simulink model "SITL"  (R2018a)
settings: Solver=VariableStepAuto  StartTime=0.0  StopTime=1000  RelTol=1e-3
settings Model: Creator=Usuario  LastModifiedBy=Usuario

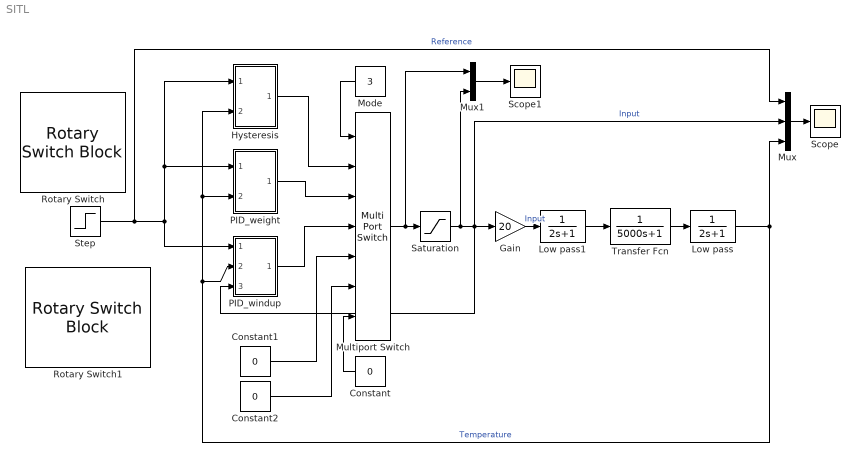
== system SITL ==
  Constant : Constant  Value=0
  Constant1 : Constant  Value=0
  Constant2 : Constant  Value=0
  Gain : Gain  Gain=20
  Hysteresis : Subsystem
  Low pass : TransferFcn  Denominator=[2 1]
  Low pass1 : TransferFcn  Denominator=[2 1]
  Mode : Constant  Value=3
  Multiport Switch : MultiPortSwitch  Inputs=5  DataPortForDefault=Additional data port
  Mux : Mux  Inputs=3
  Mux1 : Mux  Inputs=2
  PID_weight : Subsystem
  PID_windup : Subsystem
  Rotary Switch : RotarySwitchBlock  WebBlockId=48  LabelPosition=Bottom
      settings: Values={{'Off', 'Δ10', 'Δ30', 'Δ50'}, [0 10 30 50]}
  Rotary Switch1 : RotarySwitchBlock  WebBlockId=49  LabelPosition=Bottom
      settings: Values={{'Hyst', 'weight', 'windup', 'filter', 'Events'}, [1 2 3 4 5]}
  Saturation : Saturate  UpperLimit=100  LowerLimit=0
  Scope : Scope
  Scope1 : Scope
  Step : Step  Time=0  After=50  SampleTime=0
  Transfer Fcn : TransferFcn  Denominator=[5000 1]
  wires:
  Step/1 -> Mux/1, Hysteresis/1(Reference), PID_weight/1(Reference), PID_windup/1(Reference)  "Reference"
  Transfer Fcn/1 -> Low pass/1
  Mux/1 -> Scope/1
  Saturation/1 -> Mux1/2, PID_windup/3(Saturated), Mux/2, Gain/1  "Input"
  Multiport Switch/1 -> Mux1/1, Saturation/1
  Low pass/1 -> PID_windup/2(State), PID_weight/2(State), Hysteresis/2(State), Mux/3  "Temperature"
  Gain/1 -> Low pass1/1  "Input"
  Low pass1/1 -> Transfer Fcn/1
  Constant/1 -> Multiport Switch/7
  Hysteresis/1(Out) -> Multiport Switch/2
  PID_weight/1(Out) -> Multiport Switch/3
  Mode/1 -> Multiport Switch/1
  PID_windup/1(Out) -> Multiport Switch/4
  Mux1/1 -> Scope1/1
  Constant1/1 -> Multiport Switch/5
  Constant2/1 -> Multiport Switch/6

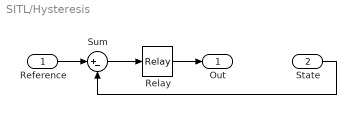
== system SITL/Hysteresis ==
  Reference : Inport
  State : Inport  Port=2
  Relay : Relay  OnSwitchValue=2  OffSwitchValue=0  OnOutputValue=100
  Sum : Sum  Inputs=|+-
  Out : Outport
  wires:
  Relay/1 -> Out/1
  State/1 -> Sum/2
  Reference/1 -> Sum/1
  Sum/1 -> Relay/1

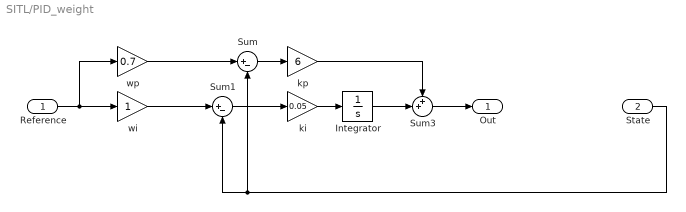
== system SITL/PID_weight ==
  Reference : Inport
  State : Inport  Port=2
  Integrator : Integrator
  Sum : Sum  Inputs=|+-
  Sum1 : Sum  Inputs=|+-
  Sum3 : Sum  Inputs=++|
  ki : Gain  Gain=0.05
  kp : Gain  Gain=6
  wi : Gain
  wp : Gain  Gain=0.7
  Out : Outport
  wires:
  kp/1 -> Sum3/1
  Sum/1 -> kp/1
  ki/1 -> Integrator/1
  State/1 -> Sum/2, Sum1/2
  Sum1/1 -> ki/1
  Sum3/1 -> Out/1
  Integrator/1 -> Sum3/2
  Reference/1 -> wp/1, wi/1
  wp/1 -> Sum/1
  wi/1 -> Sum1/1

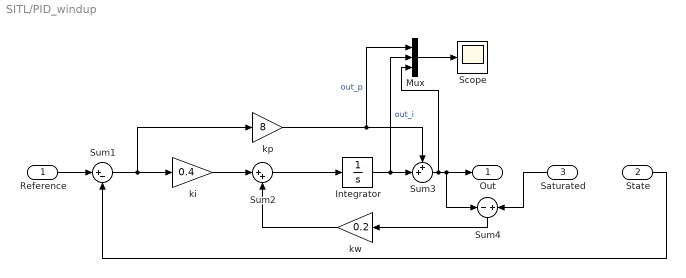
== system SITL/PID_windup ==
  Reference : Inport
  State : Inport  Port=2
  Saturated : Inport  Port=3
  Integrator : Integrator
  Mux : Mux  Inputs=3
  Scope : Scope
  Sum1 : Sum  Inputs=|+-
  Sum2 : Sum  Inputs=|++
  Sum3 : Sum  Inputs=++|
  Sum4 : Sum  Inputs=-|+
  ki : Gain  Gain=0.4
  kp : Gain  Gain=8
  kw : Gain  Gain=0.2
  Out : Outport
  wires:
  Reference/1 -> Sum1/1
  Sum3/1 -> Mux/3, Out/1, Sum4/1
  State/1 -> Sum1/2
  Sum1/1 -> ki/1, kp/1
  kp/1 -> Mux/1, Sum3/1  "out_p"
  ki/1 -> Sum2/1
  Saturated/1 -> Sum4/2
  Sum2/1 -> Integrator/1
  Sum4/1 -> kw/1
  Integrator/1 -> Mux/2, Sum3/2  "out_i"
  Mux/1 -> Scope/1
  kw/1 -> Sum2/2
